simulink model "c00002M_harness"  (R2018a)
settings: Solver=FixedStepAuto  StartTime=0.0  StopTime=300  FixedStep=0.1  RelTol=1e-3
undefined symbols (not defined in the file): A1, hmax, R1, R2, sigbuilder_block, TempThreshold
(part 3 of 14)

== system c00002M_harness/M004 ==
  note: VALUES
      | ---------------------------------
      | ControlType = 1 | 2 | 3
      | FillTank = 0 | 1
      | EmptyTank = 0 | 1
      | ManualReference between 0 and 1
      | Tempreature between 0 and 100
      | EmergencyButton = 0 | 1
      | LiquidLevel between 0 and 1 (hmax)
  note: Inputs For Tank2
  note: NAMES
      | --------------------------------------------
      | CT1 = ControlType Tank 1
      | F1 = Fill Tank 1
      | E1 = Empty Tank 1
      | MR1 = Manual Reference Tank1
      | T1 = Temperature Tank 1
      | EB1 = Emergency Button Tank 1
      | LL1 = Liquid Level 1
  note: Inputs For Tank3
  note: Inputs For Tank1
  CT1 : Inport
  MR1 : Inport  Port=2
  T1 : Inport  Port=3
  EB1 : Inport  Port=4
  CT3 : Inport  Port=5
  MR3 : Inport  Port=6
  T3 : Inport  Port=7
  EB3 : Inport  Port=8
  Tank1 : Subsystem
  Tank3 : Subsystem
  LL1 : Outport
  LL3 : Outport  Port=2
  wires:
  EB1/1 -> Tank1/4(EB1)
  Tank3/1(LL3) -> LL3/1
  MR3/1 -> Tank3/2(MR3)
  MR1/1 -> Tank1/2(MR1)
  T1/1 -> Tank1/3(T1)
  Tank1/1(LL1) -> LL1/1
  CT3/1 -> Tank3/1(CT3)
  EB3/1 -> Tank3/4(EB3)
  T3/1 -> Tank3/3(T3)
  CT1/1 -> Tank1/1(CT1)

== system c00002M_harness/M046 ==
  note: VALUES
      | ---------------------------------
      | ControlType = 1 | 2 | 3
      | FillTank = 0 | 1
      | EmptyTank = 0 | 1
      | ManualReference between 0 and 1
      | Tempreature between 0 and 100
      | EmergencyButton = 0 | 1
      | LiquidLevel between 0 and 1 (hmax)
  note: Inputs For Tank2
  note: NAMES
      | --------------------------------------------
      | CT1 = ControlType Tank 1
      | F1 = Fill Tank 1
      | E1 = Empty Tank 1
      | MR1 = Manual Reference Tank1
      | T1 = Temperature Tank 1
      | EB1 = Emergency Button Tank 1
      | LL1 = Liquid Level 1
  note: Inputs For Tank3
  note: Inputs For Tank1
  CT1 : Inport
  MR1 : Inport  Port=2
  T1 : Inport  Port=3
  EB1 : Inport  Port=4
  CT3 : Inport  Port=5
  MR3 : Inport  Port=6
  T3 : Inport  Port=7
  EB3 : Inport  Port=8
  Tank1 : Subsystem
  Tank3 : Subsystem
  LL1 : Outport
  LL3 : Outport  Port=2
  wires:
  EB1/1 -> Tank1/4(EB1)
  Tank3/1(LL3) -> LL3/1
  MR3/1 -> Tank3/2(MR3)
  MR1/1 -> Tank1/2(MR1)
  T1/1 -> Tank1/3(T1)
  Tank1/1(LL1) -> LL1/1
  CT3/1 -> Tank3/1(CT3)
  EB3/1 -> Tank3/4(EB3)
  T3/1 -> Tank3/3(T3)
  CT1/1 -> Tank1/1(CT1)

== system c00002M_harness/M047 ==
  note: VALUES
      | ---------------------------------
      | ControlType = 1 | 2 | 3
      | FillTank = 0 | 1
      | EmptyTank = 0 | 1
      | ManualReference between 0 and 1
      | Tempreature between 0 and 100
      | EmergencyButton = 0 | 1
      | LiquidLevel between 0 and 1 (hmax)
  note: Inputs For Tank2
  note: NAMES
      | --------------------------------------------
      | CT1 = ControlType Tank 1
      | F1 = Fill Tank 1
      | E1 = Empty Tank 1
      | MR1 = Manual Reference Tank1
      | T1 = Temperature Tank 1
      | EB1 = Emergency Button Tank 1
      | LL1 = Liquid Level 1
  note: Inputs For Tank3
  note: Inputs For Tank1
  CT1 : Inport
  MR1 : Inport  Port=2
  T1 : Inport  Port=3
  EB1 : Inport  Port=4
  CT3 : Inport  Port=5
  MR3 : Inport  Port=6
  T3 : Inport  Port=7
  EB3 : Inport  Port=8
  Tank1 : Subsystem
  Tank3 : Subsystem
  LL1 : Outport
  LL3 : Outport  Port=2
  wires:
  EB1/1 -> Tank1/4(EB1)
  Tank3/1(LL3) -> LL3/1
  MR3/1 -> Tank3/2(MR3)
  MR1/1 -> Tank1/2(MR1)
  T1/1 -> Tank1/3(T1)
  Tank1/1(LL1) -> LL1/1
  CT3/1 -> Tank3/1(CT3)
  EB3/1 -> Tank3/4(EB3)
  T3/1 -> Tank3/3(T3)
  CT1/1 -> Tank1/1(CT1)

== system c00002M_harness/M048 ==
  note: VALUES
      | ---------------------------------
      | ControlType = 1 | 2 | 3
      | FillTank = 0 | 1
      | EmptyTank = 0 | 1
      | ManualReference between 0 and 1
      | Tempreature between 0 and 100
      | EmergencyButton = 0 | 1
      | LiquidLevel between 0 and 1 (hmax)
  note: Inputs For Tank2
  note: NAMES
      | --------------------------------------------
      | CT1 = ControlType Tank 1
      | F1 = Fill Tank 1
      | E1 = Empty Tank 1
      | MR1 = Manual Reference Tank1
      | T1 = Temperature Tank 1
      | EB1 = Emergency Button Tank 1
      | LL1 = Liquid Level 1
  note: Inputs For Tank3
  note: Inputs For Tank1
  CT1 : Inport
  MR1 : Inport  Port=2
  T1 : Inport  Port=3
  EB1 : Inport  Port=4
  CT3 : Inport  Port=5
  MR3 : Inport  Port=6
  T3 : Inport  Port=7
  EB3 : Inport  Port=8
  Tank1 : Subsystem
  Tank3 : Subsystem
  LL1 : Outport
  LL3 : Outport  Port=2
  wires:
  EB1/1 -> Tank1/4(EB1)
  Tank3/1(LL3) -> LL3/1
  MR3/1 -> Tank3/2(MR3)
  MR1/1 -> Tank1/2(MR1)
  T1/1 -> Tank1/3(T1)
  Tank1/1(LL1) -> LL1/1
  CT3/1 -> Tank3/1(CT3)
  EB3/1 -> Tank3/4(EB3)
  T3/1 -> Tank3/3(T3)
  CT1/1 -> Tank1/1(CT1)

== system c00002M_harness/M049 ==
  note: VALUES
      | ---------------------------------
      | ControlType = 1 | 2 | 3
      | FillTank = 0 | 1
      | EmptyTank = 0 | 1
      | ManualReference between 0 and 1
      | Tempreature between 0 and 100
      | EmergencyButton = 0 | 1
      | LiquidLevel between 0 and 1 (hmax)
  note: Inputs For Tank2
  note: NAMES
      | --------------------------------------------
      | CT1 = ControlType Tank 1
      | F1 = Fill Tank 1
      | E1 = Empty Tank 1
      | MR1 = Manual Reference Tank1
      | T1 = Temperature Tank 1
      | EB1 = Emergency Button Tank 1
      | LL1 = Liquid Level 1
  note: Inputs For Tank3
  note: Inputs For Tank1
  CT1 : Inport
  MR1 : Inport  Port=2
  T1 : Inport  Port=3
  EB1 : Inport  Port=4
  CT3 : Inport  Port=5
  MR3 : Inport  Port=6
  T3 : Inport  Port=7
  EB3 : Inport  Port=8
  Tank1 : Subsystem
  Tank3 : Subsystem
  LL1 : Outport
  LL3 : Outport  Port=2
  wires:
  EB1/1 -> Tank1/4(EB1)
  Tank3/1(LL3) -> LL3/1
  MR3/1 -> Tank3/2(MR3)
  MR1/1 -> Tank1/2(MR1)
  T1/1 -> Tank1/3(T1)
  Tank1/1(LL1) -> LL1/1
  CT3/1 -> Tank3/1(CT3)
  EB3/1 -> Tank3/4(EB3)
  T3/1 -> Tank3/3(T3)
  CT1/1 -> Tank1/1(CT1)

== system c00002M_harness/M050 ==
  note: VALUES
      | ---------------------------------
      | ControlType = 1 | 2 | 3
      | FillTank = 0 | 1
      | EmptyTank = 0 | 1
      | ManualReference between 0 and 1
      | Tempreature between 0 and 100
      | EmergencyButton = 0 | 1
      | LiquidLevel between 0 and 1 (hmax)
  note: Inputs For Tank2
  note: NAMES
      | --------------------------------------------
      | CT1 = ControlType Tank 1
      | F1 = Fill Tank 1
      | E1 = Empty Tank 1
      | MR1 = Manual Reference Tank1
      | T1 = Temperature Tank 1
      | EB1 = Emergency Button Tank 1
      | LL1 = Liquid Level 1
  note: Inputs For Tank3
  note: Inputs For Tank1
  CT1 : Inport
  MR1 : Inport  Port=2
  T1 : Inport  Port=3
  EB1 : Inport  Port=4
  CT3 : Inport  Port=5
  MR3 : Inport  Port=6
  T3 : Inport  Port=7
  EB3 : Inport  Port=8
  Tank1 : Subsystem
  Tank3 : Subsystem
  LL1 : Outport
  LL3 : Outport  Port=2
  wires:
  EB1/1 -> Tank1/4(EB1)
  Tank3/1(LL3) -> LL3/1
  MR3/1 -> Tank3/2(MR3)
  MR1/1 -> Tank1/2(MR1)
  T1/1 -> Tank1/3(T1)
  Tank1/1(LL1) -> LL1/1
  CT3/1 -> Tank3/1(CT3)
  EB3/1 -> Tank3/4(EB3)
  T3/1 -> Tank3/3(T3)
  CT1/1 -> Tank1/1(CT1)

== system c00002M_harness/M051 ==
  note: VALUES
      | ---------------------------------
      | ControlType = 1 | 2 | 3
      | FillTank = 0 | 1
      | EmptyTank = 0 | 1
      | ManualReference between 0 and 1
      | Tempreature between 0 and 100
      | EmergencyButton = 0 | 1
      | LiquidLevel between 0 and 1 (hmax)
  note: Inputs For Tank2
  note: NAMES
      | --------------------------------------------
      | CT1 = ControlType Tank 1
      | F1 = Fill Tank 1
      | E1 = Empty Tank 1
      | MR1 = Manual Reference Tank1
      | T1 = Temperature Tank 1
      | EB1 = Emergency Button Tank 1
      | LL1 = Liquid Level 1
  note: Inputs For Tank3
  note: Inputs For Tank1
  CT1 : Inport
  MR1 : Inport  Port=2
  T1 : Inport  Port=3
  EB1 : Inport  Port=4
  CT3 : Inport  Port=5
  MR3 : Inport  Port=6
  T3 : Inport  Port=7
  EB3 : Inport  Port=8
  Tank1 : Subsystem
  Tank3 : Subsystem
  LL1 : Outport
  LL3 : Outport  Port=2
  wires:
  EB1/1 -> Tank1/4(EB1)
  Tank3/1(LL3) -> LL3/1
  MR3/1 -> Tank3/2(MR3)
  MR1/1 -> Tank1/2(MR1)
  T1/1 -> Tank1/3(T1)
  Tank1/1(LL1) -> LL1/1
  CT3/1 -> Tank3/1(CT3)
  EB3/1 -> Tank3/4(EB3)
  T3/1 -> Tank3/3(T3)
  CT1/1 -> Tank1/1(CT1)

== system c00002M_harness/M052 ==
  note: VALUES
      | ---------------------------------
      | ControlType = 1 | 2 | 3
      | FillTank = 0 | 1
      | EmptyTank = 0 | 1
      | ManualReference between 0 and 1
      | Tempreature between 0 and 100
      | EmergencyButton = 0 | 1
      | LiquidLevel between 0 and 1 (hmax)
  note: Inputs For Tank2
  note: NAMES
      | --------------------------------------------
      | CT1 = ControlType Tank 1
      | F1 = Fill Tank 1
      | E1 = Empty Tank 1
      | MR1 = Manual Reference Tank1
      | T1 = Temperature Tank 1
      | EB1 = Emergency Button Tank 1
      | LL1 = Liquid Level 1
  note: Inputs For Tank3
  note: Inputs For Tank1
  CT1 : Inport
  MR1 : Inport  Port=2
  T1 : Inport  Port=3
  EB1 : Inport  Port=4
  CT3 : Inport  Port=5
  MR3 : Inport  Port=6
  T3 : Inport  Port=7
  EB3 : Inport  Port=8
  Tank1 : Subsystem
  Tank3 : Subsystem
  LL1 : Outport
  LL3 : Outport  Port=2
  wires:
  EB1/1 -> Tank1/4(EB1)
  Tank3/1(LL3) -> LL3/1
  MR3/1 -> Tank3/2(MR3)
  MR1/1 -> Tank1/2(MR1)
  T1/1 -> Tank1/3(T1)
  Tank1/1(LL1) -> LL1/1
  CT3/1 -> Tank3/1(CT3)
  EB3/1 -> Tank3/4(EB3)
  T3/1 -> Tank3/3(T3)
  CT1/1 -> Tank1/1(CT1)

== system c00002M_harness/M053 ==
  note: VALUES
      | ---------------------------------
      | ControlType = 1 | 2 | 3
      | FillTank = 0 | 1
      | EmptyTank = 0 | 1
      | ManualReference between 0 and 1
      | Tempreature between 0 and 100
      | EmergencyButton = 0 | 1
      | LiquidLevel between 0 and 1 (hmax)
  note: Inputs For Tank2
  note: NAMES
      | --------------------------------------------
      | CT1 = ControlType Tank 1
      | F1 = Fill Tank 1
      | E1 = Empty Tank 1
      | MR1 = Manual Reference Tank1
      | T1 = Temperature Tank 1
      | EB1 = Emergency Button Tank 1
      | LL1 = Liquid Level 1
  note: Inputs For Tank3
  note: Inputs For Tank1
  CT1 : Inport
  MR1 : Inport  Port=2
  T1 : Inport  Port=3
  EB1 : Inport  Port=4
  CT3 : Inport  Port=5
  MR3 : Inport  Port=6
  T3 : Inport  Port=7
  EB3 : Inport  Port=8
  Tank1 : Subsystem
  Tank3 : Subsystem
  LL1 : Outport
  LL3 : Outport  Port=2
  wires:
  EB1/1 -> Tank1/4(EB1)
  Tank3/1(LL3) -> LL3/1
  MR3/1 -> Tank3/2(MR3)
  MR1/1 -> Tank1/2(MR1)
  T1/1 -> Tank1/3(T1)
  Tank1/1(LL1) -> LL1/1
  CT3/1 -> Tank3/1(CT3)
  EB3/1 -> Tank3/4(EB3)
  T3/1 -> Tank3/3(T3)
  CT1/1 -> Tank1/1(CT1)

== system c00002M_harness/M054 ==
  note: VALUES
      | ---------------------------------
      | ControlType = 1 | 2 | 3
      | FillTank = 0 | 1
      | EmptyTank = 0 | 1
      | ManualReference between 0 and 1
      | Tempreature between 0 and 100
      | EmergencyButton = 0 | 1
      | LiquidLevel between 0 and 1 (hmax)
  note: Inputs For Tank2
  note: NAMES
      | --------------------------------------------
      | CT1 = ControlType Tank 1
      | F1 = Fill Tank 1
      | E1 = Empty Tank 1
      | MR1 = Manual Reference Tank1
      | T1 = Temperature Tank 1
      | EB1 = Emergency Button Tank 1
      | LL1 = Liquid Level 1
  note: Inputs For Tank3
  note: Inputs For Tank1
  CT1 : Inport
  MR1 : Inport  Port=2
  T1 : Inport  Port=3
  EB1 : Inport  Port=4
  CT3 : Inport  Port=5
  MR3 : Inport  Port=6
  T3 : Inport  Port=7
  EB3 : Inport  Port=8
  Tank1 : Subsystem
  Tank3 : Subsystem
  LL1 : Outport
  LL3 : Outport  Port=2
  wires:
  EB1/1 -> Tank1/4(EB1)
  Tank3/1(LL3) -> LL3/1
  MR3/1 -> Tank3/2(MR3)
  MR1/1 -> Tank1/2(MR1)
  T1/1 -> Tank1/3(T1)
  Tank1/1(LL1) -> LL1/1
  CT3/1 -> Tank3/1(CT3)
  EB3/1 -> Tank3/4(EB3)
  T3/1 -> Tank3/3(T3)
  CT1/1 -> Tank1/1(CT1)

== system c00002M_harness/M055 ==
  note: VALUES
      | ---------------------------------
      | ControlType = 1 | 2 | 3
      | FillTank = 0 | 1
      | EmptyTank = 0 | 1
      | ManualReference between 0 and 1
      | Tempreature between 0 and 100
      | EmergencyButton = 0 | 1
      | LiquidLevel between 0 and 1 (hmax)
  note: Inputs For Tank2
  note: NAMES
      | --------------------------------------------
      | CT1 = ControlType Tank 1
      | F1 = Fill Tank 1
      | E1 = Empty Tank 1
      | MR1 = Manual Reference Tank1
      | T1 = Temperature Tank 1
      | EB1 = Emergency Button Tank 1
      | LL1 = Liquid Level 1
  note: Inputs For Tank3
  note: Inputs For Tank1
  CT1 : Inport
  MR1 : Inport  Port=2
  T1 : Inport  Port=3
  EB1 : Inport  Port=4
  CT3 : Inport  Port=5
  MR3 : Inport  Port=6
  T3 : Inport  Port=7
  EB3 : Inport  Port=8
  Tank1 : Subsystem
  Tank3 : Subsystem
  LL1 : Outport
  LL3 : Outport  Port=2
  wires:
  EB1/1 -> Tank1/4(EB1)
  Tank3/1(LL3) -> LL3/1
  MR3/1 -> Tank3/2(MR3)
  MR1/1 -> Tank1/2(MR1)
  T1/1 -> Tank1/3(T1)
  Tank1/1(LL1) -> LL1/1
  CT3/1 -> Tank3/1(CT3)
  EB3/1 -> Tank3/4(EB3)
  T3/1 -> Tank3/3(T3)
  CT1/1 -> Tank1/1(CT1)

== system c00002M_harness/M056 ==
  note: VALUES
      | ---------------------------------
      | ControlType = 1 | 2 | 3
      | FillTank = 0 | 1
      | EmptyTank = 0 | 1
      | ManualReference between 0 and 1
      | Tempreature between 0 and 100
      | EmergencyButton = 0 | 1
      | LiquidLevel between 0 and 1 (hmax)
  note: Inputs For Tank2
  note: NAMES
      | --------------------------------------------
      | CT1 = ControlType Tank 1
      | F1 = Fill Tank 1
      | E1 = Empty Tank 1
      | MR1 = Manual Reference Tank1
      | T1 = Temperature Tank 1
      | EB1 = Emergency Button Tank 1
      | LL1 = Liquid Level 1
  note: Inputs For Tank3
  note: Inputs For Tank1
  CT1 : Inport
  MR1 : Inport  Port=2
  T1 : Inport  Port=3
  EB1 : Inport  Port=4
  CT3 : Inport  Port=5
  MR3 : Inport  Port=6
  T3 : Inport  Port=7
  EB3 : Inport  Port=8
  Tank1 : Subsystem
  Tank3 : Subsystem
  LL1 : Outport
  LL3 : Outport  Port=2
  wires:
  EB1/1 -> Tank1/4(EB1)
  Tank3/1(LL3) -> LL3/1
  MR3/1 -> Tank3/2(MR3)
  MR1/1 -> Tank1/2(MR1)
  T1/1 -> Tank1/3(T1)
  Tank1/1(LL1) -> LL1/1
  CT3/1 -> Tank3/1(CT3)
  EB3/1 -> Tank3/4(EB3)
  T3/1 -> Tank3/3(T3)
  CT1/1 -> Tank1/1(CT1)

== system c00002M_harness/M057 ==
  note: VALUES
      | ---------------------------------
      | ControlType = 1 | 2 | 3
      | FillTank = 0 | 1
      | EmptyTank = 0 | 1
      | ManualReference between 0 and 1
      | Tempreature between 0 and 100
      | EmergencyButton = 0 | 1
      | LiquidLevel between 0 and 1 (hmax)
  note: Inputs For Tank2
  note: NAMES
      | --------------------------------------------
      | CT1 = ControlType Tank 1
      | F1 = Fill Tank 1
      | E1 = Empty Tank 1
      | MR1 = Manual Reference Tank1
      | T1 = Temperature Tank 1
      | EB1 = Emergency Button Tank 1
      | LL1 = Liquid Level 1
  note: Inputs For Tank3
  note: Inputs For Tank1
  CT1 : Inport
  MR1 : Inport  Port=2
  T1 : Inport  Port=3
  EB1 : Inport  Port=4
  CT3 : Inport  Port=5
  MR3 : Inport  Port=6
  T3 : Inport  Port=7
  EB3 : Inport  Port=8
  Tank1 : Subsystem
  Tank3 : Subsystem
  LL1 : Outport
  LL3 : Outport  Port=2
  wires:
  EB1/1 -> Tank1/4(EB1)
  Tank3/1(LL3) -> LL3/1
  MR3/1 -> Tank3/2(MR3)
  MR1/1 -> Tank1/2(MR1)
  T1/1 -> Tank1/3(T1)
  Tank1/1(LL1) -> LL1/1
  CT3/1 -> Tank3/1(CT3)
  EB3/1 -> Tank3/4(EB3)
  T3/1 -> Tank3/3(T3)
  CT1/1 -> Tank1/1(CT1)

== system c00002M_harness/M058 ==
  note: VALUES
      | ---------------------------------
      | ControlType = 1 | 2 | 3
      | FillTank = 0 | 1
      | EmptyTank = 0 | 1
      | ManualReference between 0 and 1
      | Tempreature between 0 and 100
      | EmergencyButton = 0 | 1
      | LiquidLevel between 0 and 1 (hmax)
  note: Inputs For Tank2
  note: NAMES
      | --------------------------------------------
      | CT1 = ControlType Tank 1
      | F1 = Fill Tank 1
      | E1 = Empty Tank 1
      | MR1 = Manual Reference Tank1
      | T1 = Temperature Tank 1
      | EB1 = Emergency Button Tank 1
      | LL1 = Liquid Level 1
  note: Inputs For Tank3
  note: Inputs For Tank1
  CT1 : Inport
  MR1 : Inport  Port=2
  T1 : Inport  Port=3
  EB1 : Inport  Port=4
  CT3 : Inport  Port=5
  MR3 : Inport  Port=6
  T3 : Inport  Port=7
  EB3 : Inport  Port=8
  Tank1 : Subsystem
  Tank3 : Subsystem
  LL1 : Outport
  LL3 : Outport  Port=2
  wires:
  EB1/1 -> Tank1/4(EB1)
  Tank3/1(LL3) -> LL3/1
  MR3/1 -> Tank3/2(MR3)
  MR1/1 -> Tank1/2(MR1)
  T1/1 -> Tank1/3(T1)
  Tank1/1(LL1) -> LL1/1
  CT3/1 -> Tank3/1(CT3)
  EB3/1 -> Tank3/4(EB3)
  T3/1 -> Tank3/3(T3)
  CT1/1 -> Tank1/1(CT1)

== system c00002M_harness/M059 ==
  note: VALUES
      | ---------------------------------
      | ControlType = 1 | 2 | 3
      | FillTank = 0 | 1
      | EmptyTank = 0 | 1
      | ManualReference between 0 and 1
      | Tempreature between 0 and 100
      | EmergencyButton = 0 | 1
      | LiquidLevel between 0 and 1 (hmax)
  note: Inputs For Tank2
  note: NAMES
      | --------------------------------------------
      | CT1 = ControlType Tank 1
      | F1 = Fill Tank 1
      | E1 = Empty Tank 1
      | MR1 = Manual Reference Tank1
      | T1 = Temperature Tank 1
      | EB1 = Emergency Button Tank 1
      | LL1 = Liquid Level 1
  note: Inputs For Tank3
  note: Inputs For Tank1
  CT1 : Inport
  MR1 : Inport  Port=2
  T1 : Inport  Port=3
  EB1 : Inport  Port=4
  CT3 : Inport  Port=5
  MR3 : Inport  Port=6
  T3 : Inport  Port=7
  EB3 : Inport  Port=8
  Tank1 : Subsystem
  Tank3 : Subsystem
  LL1 : Outport
  LL3 : Outport  Port=2
  wires:
  EB1/1 -> Tank1/4(EB1)
  Tank3/1(LL3) -> LL3/1
  MR3/1 -> Tank3/2(MR3)
  MR1/1 -> Tank1/2(MR1)
  T1/1 -> Tank1/3(T1)
  Tank1/1(LL1) -> LL1/1
  CT3/1 -> Tank3/1(CT3)
  EB3/1 -> Tank3/4(EB3)
  T3/1 -> Tank3/3(T3)
  CT1/1 -> Tank1/1(CT1)

== system c00002M_harness/M060 ==
  note: VALUES
      | ---------------------------------
      | ControlType = 1 | 2 | 3
      | FillTank = 0 | 1
      | EmptyTank = 0 | 1
      | ManualReference between 0 and 1
      | Tempreature between 0 and 100
      | EmergencyButton = 0 | 1
      | LiquidLevel between 0 and 1 (hmax)
  note: Inputs For Tank2
  note: NAMES
      | --------------------------------------------
      | CT1 = ControlType Tank 1
      | F1 = Fill Tank 1
      | E1 = Empty Tank 1
      | MR1 = Manual Reference Tank1
      | T1 = Temperature Tank 1
      | EB1 = Emergency Button Tank 1
      | LL1 = Liquid Level 1
  note: Inputs For Tank3
  note: Inputs For Tank1
  CT1 : Inport
  MR1 : Inport  Port=2
  T1 : Inport  Port=3
  EB1 : Inport  Port=4
  CT3 : Inport  Port=5
  MR3 : Inport  Port=6
  T3 : Inport  Port=7
  EB3 : Inport  Port=8
  Tank1 : Subsystem
  Tank3 : Subsystem
  LL1 : Outport
  LL3 : Outport  Port=2
  wires:
  EB1/1 -> Tank1/4(EB1)
  Tank3/1(LL3) -> LL3/1
  MR3/1 -> Tank3/2(MR3)
  MR1/1 -> Tank1/2(MR1)
  T1/1 -> Tank1/3(T1)
  Tank1/1(LL1) -> LL1/1
  CT3/1 -> Tank3/1(CT3)
  EB3/1 -> Tank3/4(EB3)
  T3/1 -> Tank3/3(T3)
  CT1/1 -> Tank1/1(CT1)

== system c00002M_harness/M061 ==
  note: VALUES
      | ---------------------------------
      | ControlType = 1 | 2 | 3
      | FillTank = 0 | 1
      | EmptyTank = 0 | 1
      | ManualReference between 0 and 1
      | Tempreature between 0 and 100
      | EmergencyButton = 0 | 1
      | LiquidLevel between 0 and 1 (hmax)
  note: Inputs For Tank2
  note: NAMES
      | --------------------------------------------
      | CT1 = ControlType Tank 1
      | F1 = Fill Tank 1
      | E1 = Empty Tank 1
      | MR1 = Manual Reference Tank1
      | T1 = Temperature Tank 1
      | EB1 = Emergency Button Tank 1
      | LL1 = Liquid Level 1
  note: Inputs For Tank3
  note: Inputs For Tank1
  CT1 : Inport
  MR1 : Inport  Port=2
  T1 : Inport  Port=3
  EB1 : Inport  Port=4
  CT3 : Inport  Port=5
  MR3 : Inport  Port=6
  T3 : Inport  Port=7
  EB3 : Inport  Port=8
  Tank1 : Subsystem
  Tank3 : Subsystem
  LL1 : Outport
  LL3 : Outport  Port=2
  wires:
  EB1/1 -> Tank1/4(EB1)
  Tank3/1(LL3) -> LL3/1
  MR3/1 -> Tank3/2(MR3)
  MR1/1 -> Tank1/2(MR1)
  T1/1 -> Tank1/3(T1)
  Tank1/1(LL1) -> LL1/1
  CT3/1 -> Tank3/1(CT3)
  EB3/1 -> Tank3/4(EB3)
  T3/1 -> Tank3/3(T3)
  CT1/1 -> Tank1/1(CT1)

== system c00002M_harness/M069 ==
  note: VALUES
      | ---------------------------------
      | ControlType = 1 | 2 | 3
      | FillTank = 0 | 1
      | EmptyTank = 0 | 1
      | ManualReference between 0 and 1
      | Tempreature between 0 and 100
      | EmergencyButton = 0 | 1
      | LiquidLevel between 0 and 1 (hmax)
  note: Inputs For Tank2
  note: NAMES
      | --------------------------------------------
      | CT1 = ControlType Tank 1
      | F1 = Fill Tank 1
      | E1 = Empty Tank 1
      | MR1 = Manual Reference Tank1
      | T1 = Temperature Tank 1
      | EB1 = Emergency Button Tank 1
      | LL1 = Liquid Level 1
  note: Inputs For Tank3
  note: Inputs For Tank1
  CT1 : Inport
  MR1 : Inport  Port=2
  T1 : Inport  Port=3
  EB1 : Inport  Port=4
  CT3 : Inport  Port=5
  MR3 : Inport  Port=6
  T3 : Inport  Port=7
  EB3 : Inport  Port=8
  Tank1 : Subsystem
  Tank3 : Subsystem
  LL1 : Outport
  LL3 : Outport  Port=2
  wires:
  EB1/1 -> Tank1/4(EB1)
  Tank3/1(LL3) -> LL3/1
  MR3/1 -> Tank3/2(MR3)
  MR1/1 -> Tank1/2(MR1)
  T1/1 -> Tank1/3(T1)
  Tank1/1(LL1) -> LL1/1
  CT3/1 -> Tank3/1(CT3)
  EB3/1 -> Tank3/4(EB3)
  T3/1 -> Tank3/3(T3)
  CT1/1 -> Tank1/1(CT1)

== system c00002M_harness/M070 ==
  note: VALUES
      | ---------------------------------
      | ControlType = 1 | 2 | 3
      | FillTank = 0 | 1
      | EmptyTank = 0 | 1
      | ManualReference between 0 and 1
      | Tempreature between 0 and 100
      | EmergencyButton = 0 | 1
      | LiquidLevel between 0 and 1 (hmax)
  note: Inputs For Tank2
  note: NAMES
      | --------------------------------------------
      | CT1 = ControlType Tank 1
      | F1 = Fill Tank 1
      | E1 = Empty Tank 1
      | MR1 = Manual Reference Tank1
      | T1 = Temperature Tank 1
      | EB1 = Emergency Button Tank 1
      | LL1 = Liquid Level 1
  note: Inputs For Tank3
  note: Inputs For Tank1
  CT1 : Inport
  MR1 : Inport  Port=2
  T1 : Inport  Port=3
  EB1 : Inport  Port=4
  CT3 : Inport  Port=5
  MR3 : Inport  Port=6
  T3 : Inport  Port=7
  EB3 : Inport  Port=8
  Tank1 : Subsystem
  Tank3 : Subsystem
  LL1 : Outport
  LL3 : Outport  Port=2
  wires:
  EB1/1 -> Tank1/4(EB1)
  Tank3/1(LL3) -> LL3/1
  MR3/1 -> Tank3/2(MR3)
  MR1/1 -> Tank1/2(MR1)
  T1/1 -> Tank1/3(T1)
  Tank1/1(LL1) -> LL1/1
  CT3/1 -> Tank3/1(CT3)
  EB3/1 -> Tank3/4(EB3)
  T3/1 -> Tank3/3(T3)
  CT1/1 -> Tank1/1(CT1)

== system c00002M_harness/M071 ==
  note: VALUES
      | ---------------------------------
      | ControlType = 1 | 2 | 3
      | FillTank = 0 | 1
      | EmptyTank = 0 | 1
      | ManualReference between 0 and 1
      | Tempreature between 0 and 100
      | EmergencyButton = 0 | 1
      | LiquidLevel between 0 and 1 (hmax)
  note: Inputs For Tank2
  note: NAMES
      | --------------------------------------------
      | CT1 = ControlType Tank 1
      | F1 = Fill Tank 1
      | E1 = Empty Tank 1
      | MR1 = Manual Reference Tank1
      | T1 = Temperature Tank 1
      | EB1 = Emergency Button Tank 1
      | LL1 = Liquid Level 1
  note: Inputs For Tank3
  note: Inputs For Tank1
  CT1 : Inport
  MR1 : Inport  Port=2
  T1 : Inport  Port=3
  EB1 : Inport  Port=4
  CT3 : Inport  Port=5
  MR3 : Inport  Port=6
  T3 : Inport  Port=7
  EB3 : Inport  Port=8
  Tank1 : Subsystem
  Tank3 : Subsystem
  LL1 : Outport
  LL3 : Outport  Port=2
  wires:
  EB1/1 -> Tank1/4(EB1)
  Tank3/1(LL3) -> LL3/1
  MR3/1 -> Tank3/2(MR3)
  MR1/1 -> Tank1/2(MR1)
  T1/1 -> Tank1/3(T1)
  Tank1/1(LL1) -> LL1/1
  CT3/1 -> Tank3/1(CT3)
  EB3/1 -> Tank3/4(EB3)
  T3/1 -> Tank3/3(T3)
  CT1/1 -> Tank1/1(CT1)

== system c00002M_harness/M072 ==
  note: VALUES
      | ---------------------------------
      | ControlType = 1 | 2 | 3
      | FillTank = 0 | 1
      | EmptyTank = 0 | 1
      | ManualReference between 0 and 1
      | Tempreature between 0 and 100
      | EmergencyButton = 0 | 1
      | LiquidLevel between 0 and 1 (hmax)
  note: Inputs For Tank2
  note: NAMES
      | --------------------------------------------
      | CT1 = ControlType Tank 1
      | F1 = Fill Tank 1
      | E1 = Empty Tank 1
      | MR1 = Manual Reference Tank1
      | T1 = Temperature Tank 1
      | EB1 = Emergency Button Tank 1
      | LL1 = Liquid Level 1
  note: Inputs For Tank3
  note: Inputs For Tank1
  CT1 : Inport
  MR1 : Inport  Port=2
  T1 : Inport  Port=3
  EB1 : Inport  Port=4
  CT3 : Inport  Port=5
  MR3 : Inport  Port=6
  T3 : Inport  Port=7
  EB3 : Inport  Port=8
  Tank1 : Subsystem
  Tank3 : Subsystem
  LL1 : Outport
  LL3 : Outport  Port=2
  wires:
  EB1/1 -> Tank1/4(EB1)
  Tank3/1(LL3) -> LL3/1
  MR3/1 -> Tank3/2(MR3)
  MR1/1 -> Tank1/2(MR1)
  T1/1 -> Tank1/3(T1)
  Tank1/1(LL1) -> LL1/1
  CT3/1 -> Tank3/1(CT3)
  EB3/1 -> Tank3/4(EB3)
  T3/1 -> Tank3/3(T3)
  CT1/1 -> Tank1/1(CT1)

== system c00002M_harness/M073 ==
  note: VALUES
      | ---------------------------------
      | ControlType = 1 | 2 | 3
      | FillTank = 0 | 1
      | EmptyTank = 0 | 1
      | ManualReference between 0 and 1
      | Tempreature between 0 and 100
      | EmergencyButton = 0 | 1
      | LiquidLevel between 0 and 1 (hmax)
  note: Inputs For Tank2
  note: NAMES
      | --------------------------------------------
      | CT1 = ControlType Tank 1
      | F1 = Fill Tank 1
      | E1 = Empty Tank 1
      | MR1 = Manual Reference Tank1
      | T1 = Temperature Tank 1
      | EB1 = Emergency Button Tank 1
      | LL1 = Liquid Level 1
  note: Inputs For Tank3
  note: Inputs For Tank1
  CT1 : Inport
  MR1 : Inport  Port=2
  T1 : Inport  Port=3
  EB1 : Inport  Port=4
  CT3 : Inport  Port=5
  MR3 : Inport  Port=6
  T3 : Inport  Port=7
  EB3 : Inport  Port=8
  Tank1 : Subsystem
  Tank3 : Subsystem
  LL1 : Outport
  LL3 : Outport  Port=2
  wires:
  EB1/1 -> Tank1/4(EB1)
  Tank3/1(LL3) -> LL3/1
  MR3/1 -> Tank3/2(MR3)
  MR1/1 -> Tank1/2(MR1)
  T1/1 -> Tank1/3(T1)
  Tank1/1(LL1) -> LL1/1
  CT3/1 -> Tank3/1(CT3)
  EB3/1 -> Tank3/4(EB3)
  T3/1 -> Tank3/3(T3)
  CT1/1 -> Tank1/1(CT1)

== system c00002M_harness/M074 ==
  note: VALUES
      | ---------------------------------
      | ControlType = 1 | 2 | 3
      | FillTank = 0 | 1
      | EmptyTank = 0 | 1
      | ManualReference between 0 and 1
      | Tempreature between 0 and 100
      | EmergencyButton = 0 | 1
      | LiquidLevel between 0 and 1 (hmax)
  note: Inputs For Tank2
  note: NAMES
      | --------------------------------------------
      | CT1 = ControlType Tank 1
      | F1 = Fill Tank 1
      | E1 = Empty Tank 1
      | MR1 = Manual Reference Tank1
      | T1 = Temperature Tank 1
      | EB1 = Emergency Button Tank 1
      | LL1 = Liquid Level 1
  note: Inputs For Tank3
  note: Inputs For Tank1
  CT1 : Inport
  MR1 : Inport  Port=2
  T1 : Inport  Port=3
  EB1 : Inport  Port=4
  CT3 : Inport  Port=5
  MR3 : Inport  Port=6
  T3 : Inport  Port=7
  EB3 : Inport  Port=8
  Tank1 : Subsystem
  Tank3 : Subsystem
  LL1 : Outport
  LL3 : Outport  Port=2
  wires:
  EB1/1 -> Tank1/4(EB1)
  Tank3/1(LL3) -> LL3/1
  MR3/1 -> Tank3/2(MR3)
  MR1/1 -> Tank1/2(MR1)
  T1/1 -> Tank1/3(T1)
  Tank1/1(LL1) -> LL1/1
  CT3/1 -> Tank3/1(CT3)
  EB3/1 -> Tank3/4(EB3)
  T3/1 -> Tank3/3(T3)
  CT1/1 -> Tank1/1(CT1)

== system c00002M_harness/M075 ==
  note: VALUES
      | ---------------------------------
      | ControlType = 1 | 2 | 3
      | FillTank = 0 | 1
      | EmptyTank = 0 | 1
      | ManualReference between 0 and 1
      | Tempreature between 0 and 100
      | EmergencyButton = 0 | 1
      | LiquidLevel between 0 and 1 (hmax)
  note: Inputs For Tank2
  note: NAMES
      | --------------------------------------------
      | CT1 = ControlType Tank 1
      | F1 = Fill Tank 1
      | E1 = Empty Tank 1
      | MR1 = Manual Reference Tank1
      | T1 = Temperature Tank 1
      | EB1 = Emergency Button Tank 1
      | LL1 = Liquid Level 1
  note: Inputs For Tank3
  note: Inputs For Tank1
  CT1 : Inport
  MR1 : Inport  Port=2
  T1 : Inport  Port=3
  EB1 : Inport  Port=4
  CT3 : Inport  Port=5
  MR3 : Inport  Port=6
  T3 : Inport  Port=7
  EB3 : Inport  Port=8
  Tank1 : Subsystem
  Tank3 : Subsystem
  LL1 : Outport
  LL3 : Outport  Port=2
  wires:
  EB1/1 -> Tank1/4(EB1)
  Tank3/1(LL3) -> LL3/1
  MR3/1 -> Tank3/2(MR3)
  MR1/1 -> Tank1/2(MR1)
  T1/1 -> Tank1/3(T1)
  Tank1/1(LL1) -> LL1/1
  CT3/1 -> Tank3/1(CT3)
  EB3/1 -> Tank3/4(EB3)
  T3/1 -> Tank3/3(T3)
  CT1/1 -> Tank1/1(CT1)

== system c00002M_harness/M076 ==
  note: VALUES
      | ---------------------------------
      | ControlType = 1 | 2 | 3
      | FillTank = 0 | 1
      | EmptyTank = 0 | 1
      | ManualReference between 0 and 1
      | Tempreature between 0 and 100
      | EmergencyButton = 0 | 1
      | LiquidLevel between 0 and 1 (hmax)
  note: Inputs For Tank2
  note: NAMES
      | --------------------------------------------
      | CT1 = ControlType Tank 1
      | F1 = Fill Tank 1
      | E1 = Empty Tank 1
      | MR1 = Manual Reference Tank1
      | T1 = Temperature Tank 1
      | EB1 = Emergency Button Tank 1
      | LL1 = Liquid Level 1
  note: Inputs For Tank3
  note: Inputs For Tank1
  CT1 : Inport
  MR1 : Inport  Port=2
  T1 : Inport  Port=3
  EB1 : Inport  Port=4
  CT3 : Inport  Port=5
  MR3 : Inport  Port=6
  T3 : Inport  Port=7
  EB3 : Inport  Port=8
  Tank1 : Subsystem
  Tank3 : Subsystem
  LL1 : Outport
  LL3 : Outport  Port=2
  wires:
  EB1/1 -> Tank1/4(EB1)
  Tank3/1(LL3) -> LL3/1
  MR3/1 -> Tank3/2(MR3)
  MR1/1 -> Tank1/2(MR1)
  T1/1 -> Tank1/3(T1)
  Tank1/1(LL1) -> LL1/1
  CT3/1 -> Tank3/1(CT3)
  EB3/1 -> Tank3/4(EB3)
  T3/1 -> Tank3/3(T3)
  CT1/1 -> Tank1/1(CT1)

== system c00002M_harness/M077 ==
  note: VALUES
      | ---------------------------------
      | ControlType = 1 | 2 | 3
      | FillTank = 0 | 1
      | EmptyTank = 0 | 1
      | ManualReference between 0 and 1
      | Tempreature between 0 and 100
      | EmergencyButton = 0 | 1
      | LiquidLevel between 0 and 1 (hmax)
  note: Inputs For Tank2
  note: NAMES
      | --------------------------------------------
      | CT1 = ControlType Tank 1
      | F1 = Fill Tank 1
      | E1 = Empty Tank 1
      | MR1 = Manual Reference Tank1
      | T1 = Temperature Tank 1
      | EB1 = Emergency Button Tank 1
      | LL1 = Liquid Level 1
  note: Inputs For Tank3
  note: Inputs For Tank1
  CT1 : Inport
  MR1 : Inport  Port=2
  T1 : Inport  Port=3
  EB1 : Inport  Port=4
  CT3 : Inport  Port=5
  MR3 : Inport  Port=6
  T3 : Inport  Port=7
  EB3 : Inport  Port=8
  Tank1 : Subsystem
  Tank3 : Subsystem
  LL1 : Outport
  LL3 : Outport  Port=2
  wires:
  EB1/1 -> Tank1/4(EB1)
  Tank3/1(LL3) -> LL3/1
  MR3/1 -> Tank3/2(MR3)
  MR1/1 -> Tank1/2(MR1)
  T1/1 -> Tank1/3(T1)
  Tank1/1(LL1) -> LL1/1
  CT3/1 -> Tank3/1(CT3)
  EB3/1 -> Tank3/4(EB3)
  T3/1 -> Tank3/3(T3)
  CT1/1 -> Tank1/1(CT1)

== system c00002M_harness/M078 ==
  note: VALUES
      | ---------------------------------
      | ControlType = 1 | 2 | 3
      | FillTank = 0 | 1
      | EmptyTank = 0 | 1
      | ManualReference between 0 and 1
      | Tempreature between 0 and 100
      | EmergencyButton = 0 | 1
      | LiquidLevel between 0 and 1 (hmax)
  note: Inputs For Tank2
  note: NAMES
      | --------------------------------------------
      | CT1 = ControlType Tank 1
      | F1 = Fill Tank 1
      | E1 = Empty Tank 1
      | MR1 = Manual Reference Tank1
      | T1 = Temperature Tank 1
      | EB1 = Emergency Button Tank 1
      | LL1 = Liquid Level 1
  note: Inputs For Tank3
  note: Inputs For Tank1
  CT1 : Inport
  MR1 : Inport  Port=2
  T1 : Inport  Port=3
  EB1 : Inport  Port=4
  CT3 : Inport  Port=5
  MR3 : Inport  Port=6
  T3 : Inport  Port=7
  EB3 : Inport  Port=8
  Tank1 : Subsystem
  Tank3 : Subsystem
  LL1 : Outport
  LL3 : Outport  Port=2
  wires:
  EB1/1 -> Tank1/4(EB1)
  Tank3/1(LL3) -> LL3/1
  MR3/1 -> Tank3/2(MR3)
  MR1/1 -> Tank1/2(MR1)
  T1/1 -> Tank1/3(T1)
  Tank1/1(LL1) -> LL1/1
  CT3/1 -> Tank3/1(CT3)
  EB3/1 -> Tank3/4(EB3)
  T3/1 -> Tank3/3(T3)
  CT1/1 -> Tank1/1(CT1)

== system c00002M_harness/M079 ==
  note: VALUES
      | ---------------------------------
      | ControlType = 1 | 2 | 3
      | FillTank = 0 | 1
      | EmptyTank = 0 | 1
      | ManualReference between 0 and 1
      | Tempreature between 0 and 100
      | EmergencyButton = 0 | 1
      | LiquidLevel between 0 and 1 (hmax)
  note: Inputs For Tank2
  note: NAMES
      | --------------------------------------------
      | CT1 = ControlType Tank 1
      | F1 = Fill Tank 1
      | E1 = Empty Tank 1
      | MR1 = Manual Reference Tank1
      | T1 = Temperature Tank 1
      | EB1 = Emergency Button Tank 1
      | LL1 = Liquid Level 1
  note: Inputs For Tank3
  note: Inputs For Tank1
  CT1 : Inport
  MR1 : Inport  Port=2
  T1 : Inport  Port=3
  EB1 : Inport  Port=4
  CT3 : Inport  Port=5
  MR3 : Inport  Port=6
  T3 : Inport  Port=7
  EB3 : Inport  Port=8
  Tank1 : Subsystem
  Tank3 : Subsystem
  LL1 : Outport
  LL3 : Outport  Port=2
  wires:
  EB1/1 -> Tank1/4(EB1)
  Tank3/1(LL3) -> LL3/1
  MR3/1 -> Tank3/2(MR3)
  MR1/1 -> Tank1/2(MR1)
  T1/1 -> Tank1/3(T1)
  Tank1/1(LL1) -> LL1/1
  CT3/1 -> Tank3/1(CT3)
  EB3/1 -> Tank3/4(EB3)
  T3/1 -> Tank3/3(T3)
  CT1/1 -> Tank1/1(CT1)

== system c00002M_harness/M080 ==
  note: VALUES
      | ---------------------------------
      | ControlType = 1 | 2 | 3
      | FillTank = 0 | 1
      | EmptyTank = 0 | 1
      | ManualReference between 0 and 1
      | Tempreature between 0 and 100
      | EmergencyButton = 0 | 1
      | LiquidLevel between 0 and 1 (hmax)
  note: Inputs For Tank2
  note: NAMES
      | --------------------------------------------
      | CT1 = ControlType Tank 1
      | F1 = Fill Tank 1
      | E1 = Empty Tank 1
      | MR1 = Manual Reference Tank1
      | T1 = Temperature Tank 1
      | EB1 = Emergency Button Tank 1
      | LL1 = Liquid Level 1
  note: Inputs For Tank3
  note: Inputs For Tank1
  CT1 : Inport
  MR1 : Inport  Port=2
  T1 : Inport  Port=3
  EB1 : Inport  Port=4
  CT3 : Inport  Port=5
  MR3 : Inport  Port=6
  T3 : Inport  Port=7
  EB3 : Inport  Port=8
  Tank1 : Subsystem
  Tank3 : Subsystem
  LL1 : Outport
  LL3 : Outport  Port=2
  wires:
  EB1/1 -> Tank1/4(EB1)
  Tank3/1(LL3) -> LL3/1
  MR3/1 -> Tank3/2(MR3)
  MR1/1 -> Tank1/2(MR1)
  T1/1 -> Tank1/3(T1)
  Tank1/1(LL1) -> LL1/1
  CT3/1 -> Tank3/1(CT3)
  EB3/1 -> Tank3/4(EB3)
  T3/1 -> Tank3/3(T3)
  CT1/1 -> Tank1/1(CT1)

== system c00002M_harness/M081 ==
  note: VALUES
      | ---------------------------------
      | ControlType = 1 | 2 | 3
      | FillTank = 0 | 1
      | EmptyTank = 0 | 1
      | ManualReference between 0 and 1
      | Tempreature between 0 and 100
      | EmergencyButton = 0 | 1
      | LiquidLevel between 0 and 1 (hmax)
  note: Inputs For Tank2
  note: NAMES
      | --------------------------------------------
      | CT1 = ControlType Tank 1
      | F1 = Fill Tank 1
      | E1 = Empty Tank 1
      | MR1 = Manual Reference Tank1
      | T1 = Temperature Tank 1
      | EB1 = Emergency Button Tank 1
      | LL1 = Liquid Level 1
  note: Inputs For Tank3
  note: Inputs For Tank1
  CT1 : Inport
  MR1 : Inport  Port=2
  T1 : Inport  Port=3
  EB1 : Inport  Port=4
  CT3 : Inport  Port=5
  MR3 : Inport  Port=6
  T3 : Inport  Port=7
  EB3 : Inport  Port=8
  Tank1 : Subsystem
  Tank3 : Subsystem
  LL1 : Outport
  LL3 : Outport  Port=2
  wires:
  EB1/1 -> Tank1/4(EB1)
  Tank3/1(LL3) -> LL3/1
  MR3/1 -> Tank3/2(MR3)
  MR1/1 -> Tank1/2(MR1)
  T1/1 -> Tank1/3(T1)
  Tank1/1(LL1) -> LL1/1
  CT3/1 -> Tank3/1(CT3)
  EB3/1 -> Tank3/4(EB3)
  T3/1 -> Tank3/3(T3)
  CT1/1 -> Tank1/1(CT1)

== system c00002M_harness/M082 ==
  note: VALUES
      | ---------------------------------
      | ControlType = 1 | 2 | 3
      | FillTank = 0 | 1
      | EmptyTank = 0 | 1
      | ManualReference between 0 and 1
      | Tempreature between 0 and 100
      | EmergencyButton = 0 | 1
      | LiquidLevel between 0 and 1 (hmax)
  note: Inputs For Tank2
  note: NAMES
      | --------------------------------------------
      | CT1 = ControlType Tank 1
      | F1 = Fill Tank 1
      | E1 = Empty Tank 1
      | MR1 = Manual Reference Tank1
      | T1 = Temperature Tank 1
      | EB1 = Emergency Button Tank 1
      | LL1 = Liquid Level 1
  note: Inputs For Tank3
  note: Inputs For Tank1
  CT1 : Inport
  MR1 : Inport  Port=2
  T1 : Inport  Port=3
  EB1 : Inport  Port=4
  CT3 : Inport  Port=5
  MR3 : Inport  Port=6
  T3 : Inport  Port=7
  EB3 : Inport  Port=8
  Tank1 : Subsystem
  Tank3 : Subsystem
  LL1 : Outport
  LL3 : Outport  Port=2
  wires:
  EB1/1 -> Tank1/4(EB1)
  Tank3/1(LL3) -> LL3/1
  MR3/1 -> Tank3/2(MR3)
  MR1/1 -> Tank1/2(MR1)
  T1/1 -> Tank1/3(T1)
  Tank1/1(LL1) -> LL1/1
  CT3/1 -> Tank3/1(CT3)
  EB3/1 -> Tank3/4(EB3)
  T3/1 -> Tank3/3(T3)
  CT1/1 -> Tank1/1(CT1)

== system c00002M_harness/M165 ==
  note: VALUES
      | ---------------------------------
      | ControlType = 1 | 2 | 3
      | FillTank = 0 | 1
      | EmptyTank = 0 | 1
      | ManualReference between 0 and 1
      | Tempreature between 0 and 100
      | EmergencyButton = 0 | 1
      | LiquidLevel between 0 and 1 (hmax)
  note: Inputs For Tank2
  note: NAMES
      | --------------------------------------------
      | CT1 = ControlType Tank 1
      | F1 = Fill Tank 1
      | E1 = Empty Tank 1
      | MR1 = Manual Reference Tank1
      | T1 = Temperature Tank 1
      | EB1 = Emergency Button Tank 1
      | LL1 = Liquid Level 1
  note: Inputs For Tank3
  note: Inputs For Tank1
  CT1 : Inport
  MR1 : Inport  Port=2
  T1 : Inport  Port=3
  EB1 : Inport  Port=4
  CT3 : Inport  Port=5
  MR3 : Inport  Port=6
  T3 : Inport  Port=7
  EB3 : Inport  Port=8
  Tank1 : Subsystem
  Tank3 : Subsystem
  LL1 : Outport
  LL3 : Outport  Port=2
  wires:
  EB1/1 -> Tank1/4(EB1)
  Tank3/1(LL3) -> LL3/1
  MR3/1 -> Tank3/2(MR3)
  MR1/1 -> Tank1/2(MR1)
  T1/1 -> Tank1/3(T1)
  Tank1/1(LL1) -> LL1/1
  CT3/1 -> Tank3/1(CT3)
  EB3/1 -> Tank3/4(EB3)
  T3/1 -> Tank3/3(T3)
  CT1/1 -> Tank1/1(CT1)

== system c00002M_harness/M166 ==
  note: VALUES
      | ---------------------------------
      | ControlType = 1 | 2 | 3
      | FillTank = 0 | 1
      | EmptyTank = 0 | 1
      | ManualReference between 0 and 1
      | Tempreature between 0 and 100
      | EmergencyButton = 0 | 1
      | LiquidLevel between 0 and 1 (hmax)
  note: Inputs For Tank2
  note: NAMES
      | --------------------------------------------
      | CT1 = ControlType Tank 1
      | F1 = Fill Tank 1
      | E1 = Empty Tank 1
      | MR1 = Manual Reference Tank1
      | T1 = Temperature Tank 1
      | EB1 = Emergency Button Tank 1
      | LL1 = Liquid Level 1
  note: Inputs For Tank3
  note: Inputs For Tank1
  CT1 : Inport
  MR1 : Inport  Port=2
  T1 : Inport  Port=3
  EB1 : Inport  Port=4
  CT3 : Inport  Port=5
  MR3 : Inport  Port=6
  T3 : Inport  Port=7
  EB3 : Inport  Port=8
  Tank1 : Subsystem
  Tank3 : Subsystem
  LL1 : Outport
  LL3 : Outport  Port=2
  wires:
  EB1/1 -> Tank1/4(EB1)
  Tank3/1(LL3) -> LL3/1
  MR3/1 -> Tank3/2(MR3)
  MR1/1 -> Tank1/2(MR1)
  T1/1 -> Tank1/3(T1)
  Tank1/1(LL1) -> LL1/1
  CT3/1 -> Tank3/1(CT3)
  EB3/1 -> Tank3/4(EB3)
  T3/1 -> Tank3/3(T3)
  CT1/1 -> Tank1/1(CT1)

== system c00002M_harness/M167 ==
  note: VALUES
      | ---------------------------------
      | ControlType = 1 | 2 | 3
      | FillTank = 0 | 1
      | EmptyTank = 0 | 1
      | ManualReference between 0 and 1
      | Tempreature between 0 and 100
      | EmergencyButton = 0 | 1
      | LiquidLevel between 0 and 1 (hmax)
  note: Inputs For Tank2
  note: NAMES
      | --------------------------------------------
      | CT1 = ControlType Tank 1
      | F1 = Fill Tank 1
      | E1 = Empty Tank 1
      | MR1 = Manual Reference Tank1
      | T1 = Temperature Tank 1
      | EB1 = Emergency Button Tank 1
      | LL1 = Liquid Level 1
  note: Inputs For Tank3
  note: Inputs For Tank1
  CT1 : Inport
  MR1 : Inport  Port=2
  T1 : Inport  Port=3
  EB1 : Inport  Port=4
  CT3 : Inport  Port=5
  MR3 : Inport  Port=6
  T3 : Inport  Port=7
  EB3 : Inport  Port=8
  Tank1 : Subsystem
  Tank3 : Subsystem
  LL1 : Outport
  LL3 : Outport  Port=2
  wires:
  EB1/1 -> Tank1/4(EB1)
  Tank3/1(LL3) -> LL3/1
  MR3/1 -> Tank3/2(MR3)
  MR1/1 -> Tank1/2(MR1)
  T1/1 -> Tank1/3(T1)
  Tank1/1(LL1) -> LL1/1
  CT3/1 -> Tank3/1(CT3)
  EB3/1 -> Tank3/4(EB3)
  T3/1 -> Tank3/3(T3)
  CT1/1 -> Tank1/1(CT1)

== system c00002M_harness/M168 ==
  note: VALUES
      | ---------------------------------
      | ControlType = 1 | 2 | 3
      | FillTank = 0 | 1
      | EmptyTank = 0 | 1
      | ManualReference between 0 and 1
      | Tempreature between 0 and 100
      | EmergencyButton = 0 | 1
      | LiquidLevel between 0 and 1 (hmax)
  note: Inputs For Tank2
  note: NAMES
      | --------------------------------------------
      | CT1 = ControlType Tank 1
      | F1 = Fill Tank 1
      | E1 = Empty Tank 1
      | MR1 = Manual Reference Tank1
      | T1 = Temperature Tank 1
      | EB1 = Emergency Button Tank 1
      | LL1 = Liquid Level 1
  note: Inputs For Tank3
  note: Inputs For Tank1
  CT1 : Inport
  MR1 : Inport  Port=2
  T1 : Inport  Port=3
  EB1 : Inport  Port=4
  CT3 : Inport  Port=5
  MR3 : Inport  Port=6
  T3 : Inport  Port=7
  EB3 : Inport  Port=8
  Tank1 : Subsystem
  Tank3 : Subsystem
  LL1 : Outport
  LL3 : Outport  Port=2
  wires:
  EB1/1 -> Tank1/4(EB1)
  Tank3/1(LL3) -> LL3/1
  MR3/1 -> Tank3/2(MR3)
  MR1/1 -> Tank1/2(MR1)
  T1/1 -> Tank1/3(T1)
  Tank1/1(LL1) -> LL1/1
  CT3/1 -> Tank3/1(CT3)
  EB3/1 -> Tank3/4(EB3)
  T3/1 -> Tank3/3(T3)
  CT1/1 -> Tank1/1(CT1)

== system c00002M_harness/M210 ==
  note: VALUES
      | ---------------------------------
      | ControlType = 1 | 2 | 3
      | FillTank = 0 | 1
      | EmptyTank = 0 | 1
      | ManualReference between 0 and 1
      | Tempreature between 0 and 100
      | EmergencyButton = 0 | 1
      | LiquidLevel between 0 and 1 (hmax)
  note: Inputs For Tank2
  note: NAMES
      | --------------------------------------------
      | CT1 = ControlType Tank 1
      | F1 = Fill Tank 1
      | E1 = Empty Tank 1
      | MR1 = Manual Reference Tank1
      | T1 = Temperature Tank 1
      | EB1 = Emergency Button Tank 1
      | LL1 = Liquid Level 1
  note: Inputs For Tank3
  note: Inputs For Tank1
  CT1 : Inport
  MR1 : Inport  Port=2
  T1 : Inport  Port=3
  EB1 : Inport  Port=4
  CT3 : Inport  Port=5
  MR3 : Inport  Port=6
  T3 : Inport  Port=7
  EB3 : Inport  Port=8
  Tank1 : Subsystem
  Tank3 : Subsystem
  LL1 : Outport
  LL3 : Outport  Port=2
  wires:
  EB1/1 -> Tank1/4(EB1)
  Tank3/1(LL3) -> LL3/1
  MR3/1 -> Tank3/2(MR3)
  MR1/1 -> Tank1/2(MR1)
  T1/1 -> Tank1/3(T1)
  Tank1/1(LL1) -> LL1/1
  CT3/1 -> Tank3/1(CT3)
  EB3/1 -> Tank3/4(EB3)
  T3/1 -> Tank3/3(T3)
  CT1/1 -> Tank1/1(CT1)

== system c00002M_harness/M211 ==
  note: VALUES
      | ---------------------------------
      | ControlType = 1 | 2 | 3
      | FillTank = 0 | 1
      | EmptyTank = 0 | 1
      | ManualReference between 0 and 1
      | Tempreature between 0 and 100
      | EmergencyButton = 0 | 1
      | LiquidLevel between 0 and 1 (hmax)
  note: Inputs For Tank2
  note: NAMES
      | --------------------------------------------
      | CT1 = ControlType Tank 1
      | F1 = Fill Tank 1
      | E1 = Empty Tank 1
      | MR1 = Manual Reference Tank1
      | T1 = Temperature Tank 1
      | EB1 = Emergency Button Tank 1
      | LL1 = Liquid Level 1
  note: Inputs For Tank3
  note: Inputs For Tank1
  CT1 : Inport
  MR1 : Inport  Port=2
  T1 : Inport  Port=3
  EB1 : Inport  Port=4
  CT3 : Inport  Port=5
  MR3 : Inport  Port=6
  T3 : Inport  Port=7
  EB3 : Inport  Port=8
  Tank1 : Subsystem
  Tank3 : Subsystem
  LL1 : Outport
  LL3 : Outport  Port=2
  wires:
  EB1/1 -> Tank1/4(EB1)
  Tank3/1(LL3) -> LL3/1
  MR3/1 -> Tank3/2(MR3)
  MR1/1 -> Tank1/2(MR1)
  T1/1 -> Tank1/3(T1)
  Tank1/1(LL1) -> LL1/1
  CT3/1 -> Tank3/1(CT3)
  EB3/1 -> Tank3/4(EB3)
  T3/1 -> Tank3/3(T3)
  CT1/1 -> Tank1/1(CT1)

== system c00002M_harness/M212 ==
  note: VALUES
      | ---------------------------------
      | ControlType = 1 | 2 | 3
      | FillTank = 0 | 1
      | EmptyTank = 0 | 1
      | ManualReference between 0 and 1
      | Tempreature between 0 and 100
      | EmergencyButton = 0 | 1
      | LiquidLevel between 0 and 1 (hmax)
  note: Inputs For Tank2
  note: NAMES
      | --------------------------------------------
      | CT1 = ControlType Tank 1
      | F1 = Fill Tank 1
      | E1 = Empty Tank 1
      | MR1 = Manual Reference Tank1
      | T1 = Temperature Tank 1
      | EB1 = Emergency Button Tank 1
      | LL1 = Liquid Level 1
  note: Inputs For Tank3
  note: Inputs For Tank1
  CT1 : Inport
  MR1 : Inport  Port=2
  T1 : Inport  Port=3
  EB1 : Inport  Port=4
  CT3 : Inport  Port=5
  MR3 : Inport  Port=6
  T3 : Inport  Port=7
  EB3 : Inport  Port=8
  Tank1 : Subsystem
  Tank3 : Subsystem
  LL1 : Outport
  LL3 : Outport  Port=2
  wires:
  EB1/1 -> Tank1/4(EB1)
  Tank3/1(LL3) -> LL3/1
  MR3/1 -> Tank3/2(MR3)
  MR1/1 -> Tank1/2(MR1)
  T1/1 -> Tank1/3(T1)
  Tank1/1(LL1) -> LL1/1
  CT3/1 -> Tank3/1(CT3)
  EB3/1 -> Tank3/4(EB3)
  T3/1 -> Tank3/3(T3)
  CT1/1 -> Tank1/1(CT1)

== system c00002M_harness/M213 ==
  note: VALUES
      | ---------------------------------
      | ControlType = 1 | 2 | 3
      | FillTank = 0 | 1
      | EmptyTank = 0 | 1
      | ManualReference between 0 and 1
      | Tempreature between 0 and 100
      | EmergencyButton = 0 | 1
      | LiquidLevel between 0 and 1 (hmax)
  note: Inputs For Tank2
  note: NAMES
      | --------------------------------------------
      | CT1 = ControlType Tank 1
      | F1 = Fill Tank 1
      | E1 = Empty Tank 1
      | MR1 = Manual Reference Tank1
      | T1 = Temperature Tank 1
      | EB1 = Emergency Button Tank 1
      | LL1 = Liquid Level 1
  note: Inputs For Tank3
  note: Inputs For Tank1
  CT1 : Inport
  MR1 : Inport  Port=2
  T1 : Inport  Port=3
  EB1 : Inport  Port=4
  CT3 : Inport  Port=5
  MR3 : Inport  Port=6
  T3 : Inport  Port=7
  EB3 : Inport  Port=8
  Tank1 : Subsystem
  Tank3 : Subsystem
  LL1 : Outport
  LL3 : Outport  Port=2
  wires:
  EB1/1 -> Tank1/4(EB1)
  Tank3/1(LL3) -> LL3/1
  MR3/1 -> Tank3/2(MR3)
  MR1/1 -> Tank1/2(MR1)
  T1/1 -> Tank1/3(T1)
  Tank1/1(LL1) -> LL1/1
  CT3/1 -> Tank3/1(CT3)
  EB3/1 -> Tank3/4(EB3)
  T3/1 -> Tank3/3(T3)
  CT1/1 -> Tank1/1(CT1)

== system c00002M_harness/M214 ==
  note: VALUES
      | ---------------------------------
      | ControlType = 1 | 2 | 3
      | FillTank = 0 | 1
      | EmptyTank = 0 | 1
      | ManualReference between 0 and 1
      | Tempreature between 0 and 100
      | EmergencyButton = 0 | 1
      | LiquidLevel between 0 and 1 (hmax)
  note: Inputs For Tank2
  note: NAMES
      | --------------------------------------------
      | CT1 = ControlType Tank 1
      | F1 = Fill Tank 1
      | E1 = Empty Tank 1
      | MR1 = Manual Reference Tank1
      | T1 = Temperature Tank 1
      | EB1 = Emergency Button Tank 1
      | LL1 = Liquid Level 1
  note: Inputs For Tank3
  note: Inputs For Tank1
  CT1 : Inport
  MR1 : Inport  Port=2
  T1 : Inport  Port=3
  EB1 : Inport  Port=4
  CT3 : Inport  Port=5
  MR3 : Inport  Port=6
  T3 : Inport  Port=7
  EB3 : Inport  Port=8
  Tank1 : Subsystem
  Tank3 : Subsystem
  LL1 : Outport
  LL3 : Outport  Port=2
  wires:
  EB1/1 -> Tank1/4(EB1)
  Tank3/1(LL3) -> LL3/1
  MR3/1 -> Tank3/2(MR3)
  MR1/1 -> Tank1/2(MR1)
  T1/1 -> Tank1/3(T1)
  Tank1/1(LL1) -> LL1/1
  CT3/1 -> Tank3/1(CT3)
  EB3/1 -> Tank3/4(EB3)
  T3/1 -> Tank3/3(T3)
  CT1/1 -> Tank1/1(CT1)

== system c00002M_harness/M215 ==
  note: VALUES
      | ---------------------------------
      | ControlType = 1 | 2 | 3
      | FillTank = 0 | 1
      | EmptyTank = 0 | 1
      | ManualReference between 0 and 1
      | Tempreature between 0 and 100
      | EmergencyButton = 0 | 1
      | LiquidLevel between 0 and 1 (hmax)
  note: Inputs For Tank2
  note: NAMES
      | --------------------------------------------
      | CT1 = ControlType Tank 1
      | F1 = Fill Tank 1
      | E1 = Empty Tank 1
      | MR1 = Manual Reference Tank1
      | T1 = Temperature Tank 1
      | EB1 = Emergency Button Tank 1
      | LL1 = Liquid Level 1
  note: Inputs For Tank3
  note: Inputs For Tank1
  CT1 : Inport
  MR1 : Inport  Port=2
  T1 : Inport  Port=3
  EB1 : Inport  Port=4
  CT3 : Inport  Port=5
  MR3 : Inport  Port=6
  T3 : Inport  Port=7
  EB3 : Inport  Port=8
  Tank1 : Subsystem
  Tank3 : Subsystem
  LL1 : Outport
  LL3 : Outport  Port=2
  wires:
  EB1/1 -> Tank1/4(EB1)
  Tank3/1(LL3) -> LL3/1
  MR3/1 -> Tank3/2(MR3)
  MR1/1 -> Tank1/2(MR1)
  T1/1 -> Tank1/3(T1)
  Tank1/1(LL1) -> LL1/1
  CT3/1 -> Tank3/1(CT3)
  EB3/1 -> Tank3/4(EB3)
  T3/1 -> Tank3/3(T3)
  CT1/1 -> Tank1/1(CT1)

== system c00002M_harness/M216 ==
  note: VALUES
      | ---------------------------------
      | ControlType = 1 | 2 | 3
      | FillTank = 0 | 1
      | EmptyTank = 0 | 1
      | ManualReference between 0 and 1
      | Tempreature between 0 and 100
      | EmergencyButton = 0 | 1
      | LiquidLevel between 0 and 1 (hmax)
  note: Inputs For Tank2
  note: NAMES
      | --------------------------------------------
      | CT1 = ControlType Tank 1
      | F1 = Fill Tank 1
      | E1 = Empty Tank 1
      | MR1 = Manual Reference Tank1
      | T1 = Temperature Tank 1
      | EB1 = Emergency Button Tank 1
      | LL1 = Liquid Level 1
  note: Inputs For Tank3
  note: Inputs For Tank1
  CT1 : Inport
  MR1 : Inport  Port=2
  T1 : Inport  Port=3
  EB1 : Inport  Port=4
  CT3 : Inport  Port=5
  MR3 : Inport  Port=6
  T3 : Inport  Port=7
  EB3 : Inport  Port=8
  Tank1 : Subsystem
  Tank3 : Subsystem
  LL1 : Outport
  LL3 : Outport  Port=2
  wires:
  EB1/1 -> Tank1/4(EB1)
  Tank3/1(LL3) -> LL3/1
  MR3/1 -> Tank3/2(MR3)
  MR1/1 -> Tank1/2(MR1)
  T1/1 -> Tank1/3(T1)
  Tank1/1(LL1) -> LL1/1
  CT3/1 -> Tank3/1(CT3)
  EB3/1 -> Tank3/4(EB3)
  T3/1 -> Tank3/3(T3)
  CT1/1 -> Tank1/1(CT1)

== system c00002M_harness/M217 ==
  note: VALUES
      | ---------------------------------
      | ControlType = 1 | 2 | 3
      | FillTank = 0 | 1
      | EmptyTank = 0 | 1
      | ManualReference between 0 and 1
      | Tempreature between 0 and 100
      | EmergencyButton = 0 | 1
      | LiquidLevel between 0 and 1 (hmax)
  note: Inputs For Tank2
  note: NAMES
      | --------------------------------------------
      | CT1 = ControlType Tank 1
      | F1 = Fill Tank 1
      | E1 = Empty Tank 1
      | MR1 = Manual Reference Tank1
      | T1 = Temperature Tank 1
      | EB1 = Emergency Button Tank 1
      | LL1 = Liquid Level 1
  note: Inputs For Tank3
  note: Inputs For Tank1
  CT1 : Inport
  MR1 : Inport  Port=2
  T1 : Inport  Port=3
  EB1 : Inport  Port=4
  CT3 : Inport  Port=5
  MR3 : Inport  Port=6
  T3 : Inport  Port=7
  EB3 : Inport  Port=8
  Tank1 : Subsystem
  Tank3 : Subsystem
  LL1 : Outport
  LL3 : Outport  Port=2
  wires:
  EB1/1 -> Tank1/4(EB1)
  Tank3/1(LL3) -> LL3/1
  MR3/1 -> Tank3/2(MR3)
  MR1/1 -> Tank1/2(MR1)
  T1/1 -> Tank1/3(T1)
  Tank1/1(LL1) -> LL1/1
  CT3/1 -> Tank3/1(CT3)
  EB3/1 -> Tank3/4(EB3)
  T3/1 -> Tank3/3(T3)
  CT1/1 -> Tank1/1(CT1)

== system c00002M_harness/M218 ==
  note: VALUES
      | ---------------------------------
      | ControlType = 1 | 2 | 3
      | FillTank = 0 | 1
      | EmptyTank = 0 | 1
      | ManualReference between 0 and 1
      | Tempreature between 0 and 100
      | EmergencyButton = 0 | 1
      | LiquidLevel between 0 and 1 (hmax)
  note: Inputs For Tank2
  note: NAMES
      | --------------------------------------------
      | CT1 = ControlType Tank 1
      | F1 = Fill Tank 1
      | E1 = Empty Tank 1
      | MR1 = Manual Reference Tank1
      | T1 = Temperature Tank 1
      | EB1 = Emergency Button Tank 1
      | LL1 = Liquid Level 1
  note: Inputs For Tank3
  note: Inputs For Tank1
  CT1 : Inport
  MR1 : Inport  Port=2
  T1 : Inport  Port=3
  EB1 : Inport  Port=4
  CT3 : Inport  Port=5
  MR3 : Inport  Port=6
  T3 : Inport  Port=7
  EB3 : Inport  Port=8
  Tank1 : Subsystem
  Tank3 : Subsystem
  LL1 : Outport
  LL3 : Outport  Port=2
  wires:
  EB1/1 -> Tank1/4(EB1)
  Tank3/1(LL3) -> LL3/1
  MR3/1 -> Tank3/2(MR3)
  MR1/1 -> Tank1/2(MR1)
  T1/1 -> Tank1/3(T1)
  Tank1/1(LL1) -> LL1/1
  CT3/1 -> Tank3/1(CT3)
  EB3/1 -> Tank3/4(EB3)
  T3/1 -> Tank3/3(T3)
  CT1/1 -> Tank1/1(CT1)

== system c00002M_harness/M219 ==
  note: VALUES
      | ---------------------------------
      | ControlType = 1 | 2 | 3
      | FillTank = 0 | 1
      | EmptyTank = 0 | 1
      | ManualReference between 0 and 1
      | Tempreature between 0 and 100
      | EmergencyButton = 0 | 1
      | LiquidLevel between 0 and 1 (hmax)
  note: Inputs For Tank2
  note: NAMES
      | --------------------------------------------
      | CT1 = ControlType Tank 1
      | F1 = Fill Tank 1
      | E1 = Empty Tank 1
      | MR1 = Manual Reference Tank1
      | T1 = Temperature Tank 1
      | EB1 = Emergency Button Tank 1
      | LL1 = Liquid Level 1
  note: Inputs For Tank3
  note: Inputs For Tank1
  CT1 : Inport
  MR1 : Inport  Port=2
  T1 : Inport  Port=3
  EB1 : Inport  Port=4
  CT3 : Inport  Port=5
  MR3 : Inport  Port=6
  T3 : Inport  Port=7
  EB3 : Inport  Port=8
  Tank1 : Subsystem
  Tank3 : Subsystem
  LL1 : Outport
  LL3 : Outport  Port=2
  wires:
  EB1/1 -> Tank1/4(EB1)
  Tank3/1(LL3) -> LL3/1
  MR3/1 -> Tank3/2(MR3)
  MR1/1 -> Tank1/2(MR1)
  T1/1 -> Tank1/3(T1)
  Tank1/1(LL1) -> LL1/1
  CT3/1 -> Tank3/1(CT3)
  EB3/1 -> Tank3/4(EB3)
  T3/1 -> Tank3/3(T3)
  CT1/1 -> Tank1/1(CT1)

== system c00002M_harness/M220 ==
  note: VALUES
      | ---------------------------------
      | ControlType = 1 | 2 | 3
      | FillTank = 0 | 1
      | EmptyTank = 0 | 1
      | ManualReference between 0 and 1
      | Tempreature between 0 and 100
      | EmergencyButton = 0 | 1
      | LiquidLevel between 0 and 1 (hmax)
  note: Inputs For Tank2
  note: NAMES
      | --------------------------------------------
      | CT1 = ControlType Tank 1
      | F1 = Fill Tank 1
      | E1 = Empty Tank 1
      | MR1 = Manual Reference Tank1
      | T1 = Temperature Tank 1
      | EB1 = Emergency Button Tank 1
      | LL1 = Liquid Level 1
  note: Inputs For Tank3
  note: Inputs For Tank1
  CT1 : Inport
  MR1 : Inport  Port=2
  T1 : Inport  Port=3
  EB1 : Inport  Port=4
  CT3 : Inport  Port=5
  MR3 : Inport  Port=6
  T3 : Inport  Port=7
  EB3 : Inport  Port=8
  Tank1 : Subsystem
  Tank3 : Subsystem
  LL1 : Outport
  LL3 : Outport  Port=2
  wires:
  EB1/1 -> Tank1/4(EB1)
  Tank3/1(LL3) -> LL3/1
  MR3/1 -> Tank3/2(MR3)
  MR1/1 -> Tank1/2(MR1)
  T1/1 -> Tank1/3(T1)
  Tank1/1(LL1) -> LL1/1
  CT3/1 -> Tank3/1(CT3)
  EB3/1 -> Tank3/4(EB3)
  T3/1 -> Tank3/3(T3)
  CT1/1 -> Tank1/1(CT1)
